simulink library "amg_sense_light_lib"  (R2015b)
settings: Solver=ode45  StartTime=0.0  StopTime=10.0  RelTol=1e-3
libraries: simulink x37, stm32f4_i2c_lib x3, waijung_soft_i2c_lib x3, waijung_customcode x1
(part 1 of 2)
settings Model: Creator=Krisada  LastModifiedBy=Aimagin
settings DataIOCC: SaveFormat=Array  SignalLoggingSaveFormat=ModelDataLogs
settings OptimizationCC: ExpressionDepthLimit=2147483647
settings DebuggingCC: UnderspecifiedInitializationDetection=Classic  MergeDetectMultiDrivingBlocksExec=none  SolverPrmCheckMsg=warning  FcnCallInpInsideContextMsg=UseLocalSettings  StateNameClashWarn=warning  StrictBusMsg=Warning
settings HardwareCC: ProdBitPerPointer=32  ProdLargestAtomicFloat=None  ProdIntDivRoundTo=Undefined  ProdEndianess=Unspecified  ProdWordSize=32  ProdHWDeviceType=32-bit Generic
settings GRTTargetCC: CombineOutputUpdateFcns=off  GRTInterface=on
settings ConfigComp: CovModelRefEnable=Off

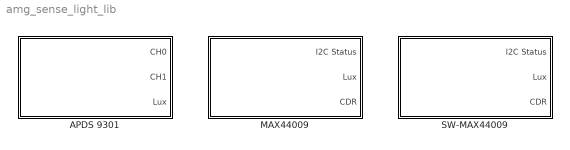
== system amg_sense_light_lib ==
  APDS 9301 : Subsystem  mask(stm32f4_i2c_sensors){module=1, slvaddr=hex2dec('72'), outputlabel={'CH0','CH1','Lux'}, sensorname=STM32F4\naMG Sense - Light, sampletime=0.5}
      mask prompts: module "I2C Module"; slvaddr "I2C Slave Address"; outputlabel "Output label"; sensorname "Sensor name"; sampletime "Sample time (sec)"
      mask help:
      | aMG Sense - Light
      |
      | Note: Require I2C Setup block for the selected I2C module.
      mask init:
      | stm32f4_i2c_sensors_callback('init');
      mask TypeOptions module: 1 | 2 | 3
      mask Callback module: stm32f4_i2c_sensors_callback('module');
      mask Display: text(0.5, 0.5, 'STM32F4\naMG Sense - Light','ver','middle','hor','center');port_label('output', 1,'CH0');port_label('output', 2,'CH1');port_label('output', 3,'Lux');
  MAX44009 : Subsystem  mask(stm32f4_i2c_sensors){module=1, slvaddr=hex2dec('94'), outputlabel={'I2C Status','Lux','CDR'}, sensorname=STM32F4\naMG Sense - Light\nMAX44009, sampletime=1}
      mask prompts: module "I2C Module"; slvaddr "I2C Slave Address"; outputlabel "Output label"; sensorname "Sensor name"; sampletime "Sample time (sec)"
      mask help:
      | aMG Sense - Light
      |
      | I2C Status:
      |  0 - Success
      |  1 - NAK
      |  2 - Timeout
      |  3 - Combined error, NAK+Timeout
      |
      | Note: Require I2C Setup block for the selected I2C module.
      mask init:
      | stm32f4_i2c_sensors_callback('init');
      mask TypeOptions module: 1 | 2 | 3
      mask Callback module: stm32f4_i2c_sensors_callback('module');
      mask Display: text(0.5, 0.5, 'STM32F4\naMG Sense - Light\nMAX44009','ver','middle','hor','center');port_label('output', 1,'I2C Status');port_label('output', 2,'Lux');port_label('output', 3,'CDR');
  SW-MAX44009 : Subsystem  mask(waijung_soft_i2c_sensors){module=1, slvaddr=hex2dec('94'), outputlabel={'I2C Status','Lux','CDR'}, sensorname=Soft-I2C\naMG Sense - Light\nMAX44009, sampletime=1}
      mask prompts: module "I2C Module"; slvaddr "I2C Slave Address"; outputlabel "Output label"; sensorname "Sensor name"; sampletime "Sample time (sec)"
      mask help:
      | aMG Sense - Light
      |
      | I2C Status:
      |  0 - Success
      |  1 - NAK
      |  2 - Timeout
      |  3 - Combined error, NAK+Timeout
      |
      | Note: Require I2C Setup block for the selected I2C module.
      mask init:
      | waijung_soft_i2c_sensors_callback('init');
      mask TypeOptions module: 1 | 2 | 3
      mask Callback module: waijung_soft_i2c_sensors_callback('module');
      mask Display: text(0.5, 0.5, 'Soft-I2C\naMG Sense - Light\nMAX44009','ver','middle','hor','center');port_label('output', 1,'I2C Status');port_label('output', 2,'Lux');port_label('output', 3,'CDR');

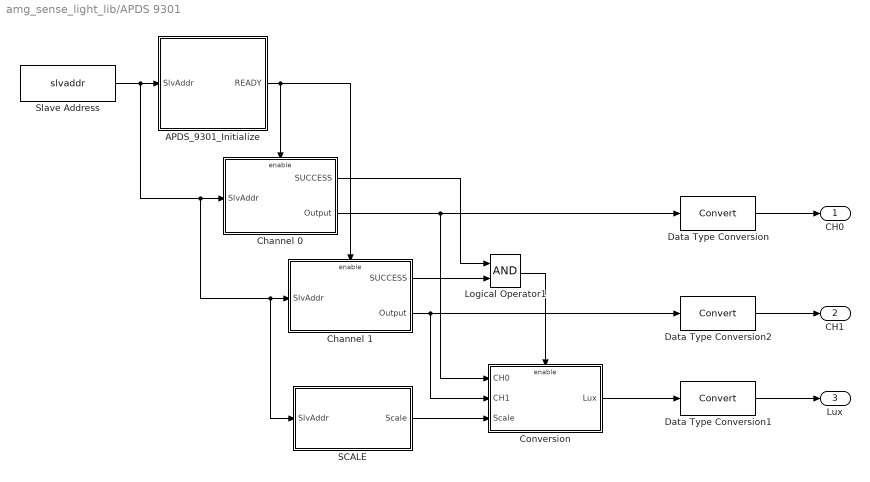
== system amg_sense_light_lib/APDS 9301 ==
  APDS_9301_Initialize : Subsystem
  Channel 0 : Subsystem
  Channel 1 : Subsystem
  Conversion : Subsystem
  Data Type Conversion : DataTypeConversion
  Data Type Conversion1 : DataTypeConversion
  Data Type Conversion2 : DataTypeConversion
  Logical Operator1 : Logic  AllPortsSameDT=off  OutDataTypeStr=boolean
  SCALE : Subsystem
  Slave Address : Constant  Value=slvaddr  OutDataTypeStr=uint8  SampleTime=sampletime
  CH0 : Outport
  CH1 : Outport  Port=2
  Lux : Outport  Port=3
  wires:
  Data Type Conversion/1 -> CH0/1
  Data Type Conversion2/1 -> CH1/1
  Data Type Conversion1/1 -> Lux/1
  Slave Address/1 -> APDS_9301_Initialize/1(SlvAddr), Channel 0/1(SlvAddr), Channel 1/1(SlvAddr), SCALE/1(SlvAddr)
  APDS_9301_Initialize/1(READY) -> Channel 0/Enable, Channel 1/Enable
  Channel 0/2(Output) -> Conversion/1(CH0), Data Type Conversion/1
  Channel 1/1(SUCCESS) -> Logical Operator1/2
  Channel 0/1(SUCCESS) -> Logical Operator1/1
  Conversion/1(Lux) -> Data Type Conversion1/1
  Channel 1/2(Output) -> Conversion/2(CH1), Data Type Conversion2/1
  Logical Operator1/1 -> Conversion/Enable
  SCALE/1(Scale) -> Conversion/3(Scale)

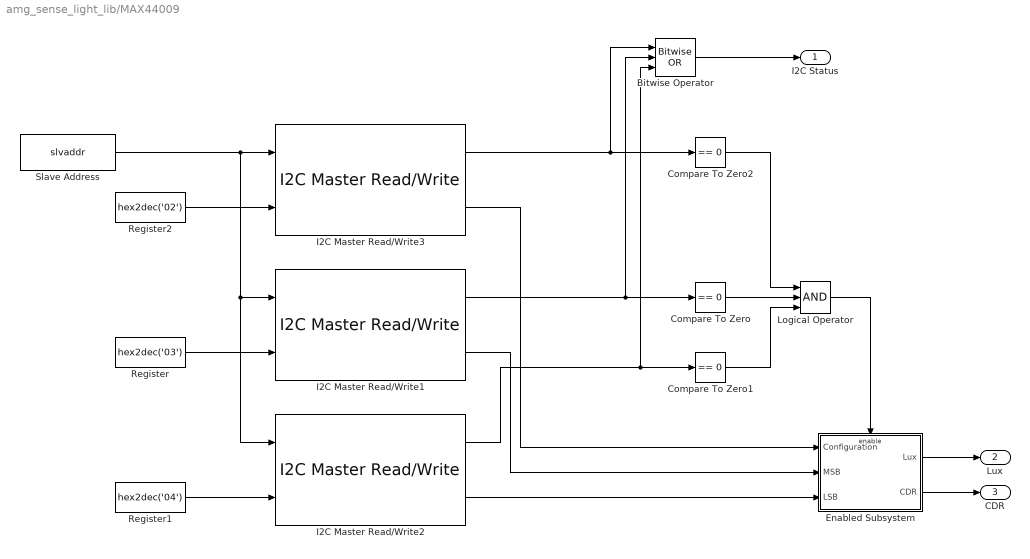
== system amg_sense_light_lib/MAX44009 ==
  Bitwise Operator : simulink/Logic and Bit Operations/Bitwise Operator  logicop=OR  UseBitMask=off  NumInputPorts=3  BitMask=bin2dec('11011001')  BitMaskRealWorld=Stored Integer
  Compare To Zero : simulink/Logic and Bit Operations/Compare To Zero  SystemSampleTime=-1  relop===  LogicOutDataTypeMode=uint8  ZeroCross=off
  Compare To Zero1 : simulink/Logic and Bit Operations/Compare To Zero  SystemSampleTime=-1  relop===  LogicOutDataTypeMode=uint8  ZeroCross=off
  Compare To Zero2 : simulink/Logic and Bit Operations/Compare To Zero  SystemSampleTime=-1  relop===  LogicOutDataTypeMode=uint8  ZeroCross=off
  Enabled Subsystem : Subsystem  TreatAsAtomicUnit=on
  I2C Master Read/Write1 : stm32f4_i2c_lib/I2C Master Read//Write  configuration=Transaction  module=1  lastmodule=3  transfer=Blocking  dutycycle=TLow/THigh = 2  clkspeed=400  timeout=25  writecount=1  readcount=1  sdapin=C9  sclpin=A8  waitwritetime=0  forcestop=off  inputtypearray=[2 3 3]  outputtypearray=[2 3 3]  confstr="[\"C\",\"9\",\"A\",\"8\",\"1\",\"1\",\"6\",\"0\",\"I2C_DutyCycle_2\",\"0\",\"off\"]"  sampletime=-1  sampletimestr=1  blockid=MAX44009I2CMasterReadWrite1
  I2C Master Read/Write2 : stm32f4_i2c_lib/I2C Master Read//Write  configuration=Transaction  module=1  lastmodule=3  transfer=Blocking  dutycycle=TLow/THigh = 2  clkspeed=400  timeout=25  writecount=1  readcount=1  sdapin=C9  sclpin=A8  waitwritetime=0  forcestop=off  inputtypearray=[2 3 3]  outputtypearray=[2 3 3]  confstr="[\"C\",\"9\",\"A\",\"8\",\"1\",\"1\",\"6\",\"0\",\"I2C_DutyCycle_2\",\"0\",\"off\"]"  sampletime=-1  sampletimestr=1  blockid=MAX44009I2CMasterReadWrite2
  I2C Master Read/Write3 : stm32f4_i2c_lib/I2C Master Read//Write  configuration=Transaction  module=1  lastmodule=3  transfer=Blocking  dutycycle=TLow/THigh = 2  clkspeed=400  timeout=25  writecount=1  readcount=1  sdapin=C9  sclpin=A8  waitwritetime=0  forcestop=off  inputtypearray=[2 3 3]  outputtypearray=[2 3 3]  confstr="[\"C\",\"9\",\"A\",\"8\",\"1\",\"1\",\"6\",\"0\",\"I2C_DutyCycle_2\",\"0\",\"off\"]"  sampletime=-1  sampletimestr=1  blockid=MAX44009I2CMasterReadWrite3
  Logical Operator : Logic  Inputs=3  AllPortsSameDT=off  OutDataTypeStr=boolean
  Register : Constant  Value=hex2dec('03')  OutDataTypeStr=uint8
  Register1 : Constant  Value=hex2dec('04')  OutDataTypeStr=uint8
  Register2 : Constant  Value=hex2dec('02')  OutDataTypeStr=uint8
  Slave Address : Constant  Value=slvaddr  OutDataTypeStr=uint8  SampleTime=sampletime
  I2C Status : Outport
  Lux : Outport  Port=2
  CDR : Outport  Port=3
  wires:
  I2C Master Read/Write3/2 -> Enabled Subsystem/1(Configuration)
  Compare To Zero1/1 -> Logical Operator/3
  Compare To Zero2/1 -> Logical Operator/1
  Compare To Zero/1 -> Logical Operator/2
  I2C Master Read/Write3/1 -> Compare To Zero2/1, Bitwise Operator/1
  Register2/1 -> I2C Master Read/Write3/2
  I2C Master Read/Write2/2 -> Enabled Subsystem/3(LSB)
  I2C Master Read/Write1/2 -> Enabled Subsystem/2(MSB)
  Logical Operator/1 -> Enabled Subsystem/Enable
  I2C Master Read/Write2/1 -> Compare To Zero1/1, Bitwise Operator/3
  Register1/1 -> I2C Master Read/Write2/2
  Slave Address/1 -> I2C Master Read/Write3/1, I2C Master Read/Write2/1, I2C Master Read/Write1/1
  Register/1 -> I2C Master Read/Write1/2
  I2C Master Read/Write1/1 -> Compare To Zero/1, Bitwise Operator/2
  Enabled Subsystem/1(Lux) -> Lux/1
  Enabled Subsystem/2(CDR) -> CDR/1
  Bitwise Operator/1 -> I2C Status/1

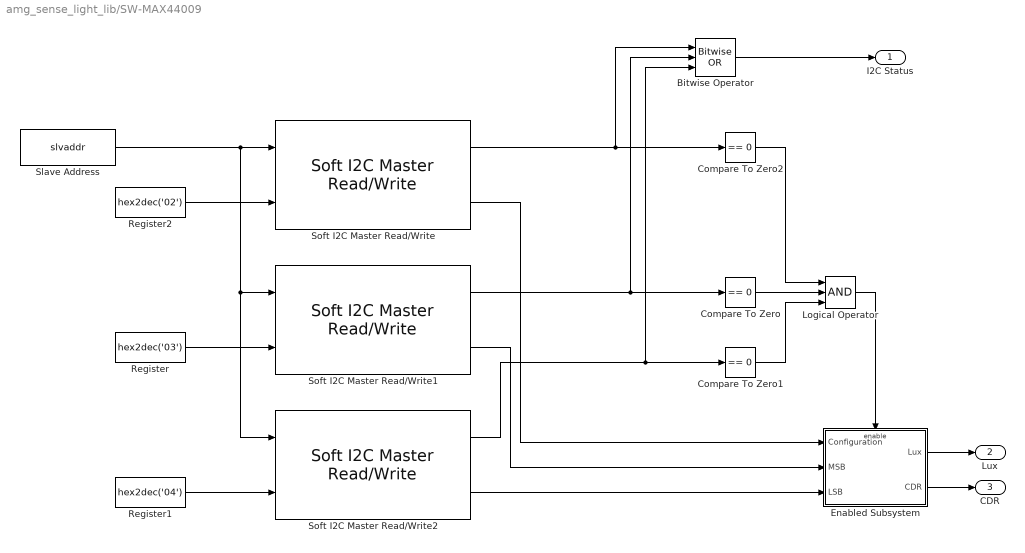
== system amg_sense_light_lib/SW-MAX44009 ==
  Bitwise Operator : simulink/Logic and Bit Operations/Bitwise Operator  logicop=OR  UseBitMask=off  NumInputPorts=3  BitMask=bin2dec('11011001')  BitMaskRealWorld=Stored Integer
  Compare To Zero : simulink/Logic and Bit Operations/Compare To Zero  SystemSampleTime=-1  relop===  LogicOutDataTypeMode=uint8  ZeroCross=off
  Compare To Zero1 : simulink/Logic and Bit Operations/Compare To Zero  SystemSampleTime=-1  relop===  LogicOutDataTypeMode=uint8  ZeroCross=off
  Compare To Zero2 : simulink/Logic and Bit Operations/Compare To Zero  SystemSampleTime=-1  relop===  LogicOutDataTypeMode=uint8  ZeroCross=off
  Enabled Subsystem : Subsystem  TreatAsAtomicUnit=on
  Logical Operator : Logic  Inputs=3  AllPortsSameDT=off  OutDataTypeStr=boolean
  Register : Constant  Value=hex2dec('03')  OutDataTypeStr=uint8
  Register1 : Constant  Value=hex2dec('04')  OutDataTypeStr=uint8
  Register2 : Constant  Value=hex2dec('02')  OutDataTypeStr=uint8
  Slave Address : Constant  Value=slvaddr  OutDataTypeStr=uint8  SampleTime=sampletime
  Soft I2C Master Read/Write : waijung_soft_i2c_lib/Soft I2C Master Read//Write  conf=ReadWrite  targetname=0  module=1  transfer=Blocking  clk=100  timeout=25  sdapins={'A4','A6'}  sclpins='A5'  writecount=1  readcount=1  waittime=0  forcestop=off  portpinstr=0  sampletime=inf  blockid=SWMAX44009SoftI2CMasterReadWrite  inputporttype=[3 3]  inputportwidth=[]  inputportlabel={'SlvAddr' 'Wr0 (uint8)'}  outputporttype=[3 3]  outputportwidth=[1 1]  outputportlabel={'Status' 'Rd0 (uint8)'}  compat=0  optionstring=[]
  Soft I2C Master Read/Write1 : waijung_soft_i2c_lib/Soft I2C Master Read//Write  conf=ReadWrite  targetname=0  module=1  transfer=Blocking  clk=100  timeout=25  sdapins={'A4','A6'}  sclpins='A5'  writecount=1  readcount=1  waittime=0  forcestop=off  portpinstr=0  sampletime=inf  blockid=SWMAX44009SoftI2CMasterReadWrite1  inputporttype=[3 3]  inputportwidth=[]  inputportlabel={'SlvAddr' 'Wr0 (uint8)'}  outputporttype=[3 3]  outputportwidth=[1 1]  outputportlabel={'Status' 'Rd0 (uint8)'}  compat=0  optionstring=[]
  Soft I2C Master Read/Write2 : waijung_soft_i2c_lib/Soft I2C Master Read//Write  conf=ReadWrite  targetname=0  module=1  transfer=Blocking  clk=100  timeout=25  sdapins={'A4','A6'}  sclpins='A5'  writecount=1  readcount=1  waittime=0  forcestop=off  portpinstr=0  sampletime=inf  blockid=SWMAX44009SoftI2CMasterReadWrite2  inputporttype=[3 3]  inputportwidth=[]  inputportlabel={'SlvAddr' 'Wr0 (uint8)'}  outputporttype=[3 3]  outputportwidth=[1 1]  outputportlabel={'Status' 'Rd0 (uint8)'}  compat=0  optionstring=[]
  I2C Status : Outport
  Lux : Outport  Port=2
  CDR : Outport  Port=3
  wires:
  Enabled Subsystem/2(CDR) -> CDR/1
  Enabled Subsystem/1(Lux) -> Lux/1
  Soft I2C Master Read/Write1/1 -> Compare To Zero/1, Bitwise Operator/2
  Register/1 -> Soft I2C Master Read/Write1/2
  Slave Address/1 -> Soft I2C Master Read/Write1/1, Soft I2C Master Read/Write2/1, Soft I2C Master Read/Write/1
  Register1/1 -> Soft I2C Master Read/Write2/2
  Soft I2C Master Read/Write2/1 -> Compare To Zero1/1, Bitwise Operator/3
  Logical Operator/1 -> Enabled Subsystem/Enable
  Soft I2C Master Read/Write1/2 -> Enabled Subsystem/2(MSB)
  Soft I2C Master Read/Write2/2 -> Enabled Subsystem/3(LSB)
  Register2/1 -> Soft I2C Master Read/Write/2
  Soft I2C Master Read/Write/1 -> Compare To Zero2/1, Bitwise Operator/1
  Compare To Zero/1 -> Logical Operator/2
  Compare To Zero2/1 -> Logical Operator/1
  Compare To Zero1/1 -> Logical Operator/3
  Soft I2C Master Read/Write/2 -> Enabled Subsystem/1(Configuration)
  Bitwise Operator/1 -> I2C Status/1

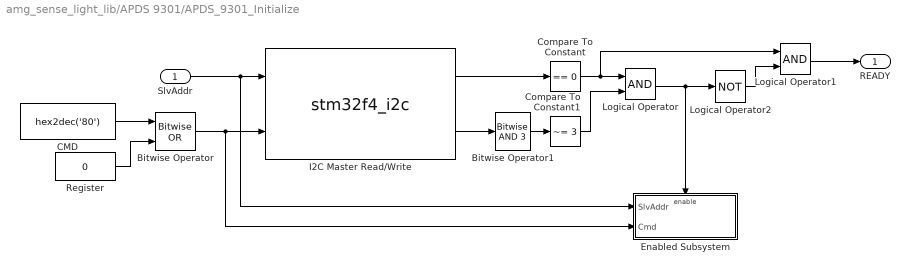
== system amg_sense_light_lib/APDS 9301/APDS_9301_Initialize ==
  SlvAddr : Inport
  Bitwise Operator : simulink/Logic and Bit Operations/Bitwise Operator  logicop=OR  UseBitMask=off  NumInputPorts=2  BitMask=bin2dec('11011001')  BitMaskRealWorld=Stored Integer
  Bitwise Operator1 : simulink/Logic and Bit Operations/Bitwise Operator  logicop=AND  UseBitMask=on  BitMask=3  BitMaskRealWorld=Stored Integer
  CMD : Constant  Value=hex2dec('80')  OutDataTypeStr=uint8
  Compare To Constant : simulink/Logic and Bit Operations/Compare To Constant  SystemSampleTime=-1  relop===  const=0  LogicOutDataTypeMode=uint8  ZeroCross=off
  Compare To Constant1 : simulink/Logic and Bit Operations/Compare To Constant  SystemSampleTime=-1  relop=~=  const=3  LogicOutDataTypeMode=uint8  ZeroCross=off
  Enabled Subsystem : Subsystem  TreatAsAtomicUnit=on
  I2C Master Read/Write : S-Function  FunctionName=stm32f4_i2c  Parameters=configuration,module,transfer,clkspeed,timeout,sdapin,sclpin,writecount,readcount,inputtypearray,outputtypearray,confstr,sampletime,sampletimestr,blockid  SFunctionDeploymentMode=off  EnableBusSupport=off  mask(stm32f4_i2c){configuration=Transaction, module=1, lastmodule=3, transfer=Blocking, dutycycle=TLow/THigh = 2, clkspeed=400, timeout=25, writecount=1, readcount=1, sdapin=C9, sclpin=A8, waitwritetime=0, inputtypearray=[2 3 3], outputtypearray=[2 3 3], confstr=["C","9","A","8","1","1","6","0","I2C_DutyCycle_2","0","off"], sampletime=-1, sampletimestr=1, blockid=APDS_9301_InitializeI2CMasterReadWrite}
      mask prompts: module "I2C Module"; lastmodule "Last module"; transfer "Transfer mode"; dutycycle "Duty cycle in fast mode"; clkspeed "Clock speed (kHz)"; timeout "Timeout (ms)"; writecount "Bytes write count"; readcount "Bytes read count"; sdapin "SDA pin"; sclpin "SCL pin"; waitwritetime "Wait write time (ms), default is 0"; inputtypearray "Input type array"; outputtypearray "Output type array"; confstr "Configuration string"; sampletime "Sample time (sec)"; sampletimestr "Compiled sample time (sec) in string"
      mask init:
      | stm32f4_i2c_callback('init');
      mask Help: web(fullfile(waijungdocroot,'stm32f4_i2c_readwrite.htm'), '-browser')
      mask TypeOptions configuration: Setup | Transaction
      mask Callback configuration: stm32f4_i2c_callback('configuration');
      mask TypeOptions module: 1 | 2 | 3
      mask Callback module: stm32f4_i2c_callback('module');
      mask TypeOptions transfer: Blocking | Non-blocking
      mask TypeOptions dutycycle: TLow/THigh = 16/9 | TLow/THigh = 2
      mask Callback dutycycle: stm32f4_i2c_callback('dutycycle');
      mask Callback writecount: stm32f4_i2c_callback('writecount');
      mask Callback readcount: stm32f4_i2c_callback('readcount');
      mask TypeOptions sdapin: - | C9
      mask Callback sdapin: stm32f4_i2c_callback('sdapin');
      mask TypeOptions sclpin: - | A8
      mask Callback sclpin: stm32f4_i2c_callback('sclpin');
      mask Callback confstr: stm32f4_i2c_callback('confstr');
      mask Callback sampletime: stm32f4_i2c_callback('sampletime');
      mask Callback sampletimestr: stm32f4_i2c_callback('sampletimestr');
      mask Callback blockid: stm32f4_i2c_callback('blockid');
      mask Display: text(0.5, 0.5, 'Module: I2C1\nTransfer: Blocking\nWrite: 1 bytes\nRead: 1 bytes\nTs (sec): 1','ver','middle','hor','center');port_label('input', 1,'SlvAddr');port_label('input', 2,'Wr0 (uint8)');port_label('output', 1,'Status');port_label('output', 2,'Rd0 (uint8)');
  Logical Operator : Logic  AllPortsSameDT=off  OutDataTypeStr=boolean
  Logical Operator1 : Logic  AllPortsSameDT=off  OutDataTypeStr=boolean
  Logical Operator2 : Logic  Operator=NOT  AllPortsSameDT=off  OutDataTypeStr=boolean
  Register : Constant  Value=0  OutDataTypeStr=uint8
  READY : Outport
  wires:
  SlvAddr/1 -> I2C Master Read/Write/1, Enabled Subsystem/1(SlvAddr)
  Bitwise Operator/1 -> I2C Master Read/Write/2, Enabled Subsystem/2(Cmd)
  CMD/1 -> Bitwise Operator/1
  I2C Master Read/Write/1 -> Compare To Constant/1
  I2C Master Read/Write/2 -> Bitwise Operator1/1
  Compare To Constant/1 -> Logical Operator/1, Logical Operator1/1
  Compare To Constant1/1 -> Logical Operator/2
  Logical Operator/1 -> Enabled Subsystem/Enable, Logical Operator2/1
  Register/1 -> Bitwise Operator/2
  Bitwise Operator1/1 -> Compare To Constant1/1
  Logical Operator2/1 -> Logical Operator1/2
  Logical Operator1/1 -> READY/1

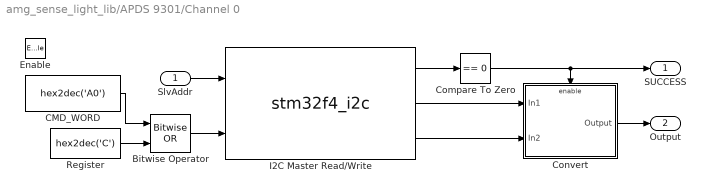
== system amg_sense_light_lib/APDS 9301/Channel 0 ==
  SlvAddr : Inport
  Enable : EnablePort  PropagateVarSize=During execution
  Bitwise Operator : simulink/Logic and Bit Operations/Bitwise Operator  logicop=OR  UseBitMask=off  NumInputPorts=2  BitMask=bin2dec('11011001')  BitMaskRealWorld=Stored Integer
  CMD_WORD : Constant  Value=hex2dec('A0')  OutDataTypeStr=uint8
  Compare To Zero : simulink/Logic and Bit Operations/Compare To Zero  SystemSampleTime=-1  relop===  LogicOutDataTypeMode=uint8  ZeroCross=off
  Convert : Subsystem
  I2C Master Read/Write : S-Function  FunctionName=stm32f4_i2c  Parameters=configuration,module,transfer,clkspeed,timeout,sdapin,sclpin,writecount,readcount,inputtypearray,outputtypearray,confstr,sampletime,sampletimestr,blockid  SFunctionDeploymentMode=off  EnableBusSupport=off  mask(stm32f4_i2c){configuration=Transaction, module=1, lastmodule=3, transfer=Blocking, dutycycle=TLow/THigh = 2, clkspeed=400, timeout=25, writecount=1, readcount=2, sdapin=C9, sclpin=A8, waitwritetime=0, inputtypearray=[2 3 3], outputtypearray=[3 3 3 3], confstr=["C","9","A","8","1","1","6","0","I2C_DutyCycle_2","0","off"], sampletime=-1, sampletimestr=1, blockid=Channel0I2CMasterReadWrite}
      mask prompts: module "I2C Module"; lastmodule "Last module"; transfer "Transfer mode"; dutycycle "Duty cycle in fast mode"; clkspeed "Clock speed (kHz)"; timeout "Timeout (ms)"; writecount "Bytes write count"; readcount "Bytes read count"; sdapin "SDA pin"; sclpin "SCL pin"; waitwritetime "Wait write time (ms), default is 0"; inputtypearray "Input type array"; outputtypearray "Output type array"; confstr "Configuration string"; sampletime "Sample time (sec)"; sampletimestr "Compiled sample time (sec) in string"
      mask init:
      | stm32f4_i2c_callback('init');
      mask Help: web(fullfile(waijungdocroot,'stm32f4_i2c_readwrite.htm'), '-browser')
      mask TypeOptions configuration: Setup | Transaction
      mask Callback configuration: stm32f4_i2c_callback('configuration');
      mask TypeOptions module: 1 | 2 | 3
      mask Callback module: stm32f4_i2c_callback('module');
      mask TypeOptions transfer: Blocking | Non-blocking
      mask TypeOptions dutycycle: TLow/THigh = 16/9 | TLow/THigh = 2
      mask Callback dutycycle: stm32f4_i2c_callback('dutycycle');
      mask Callback writecount: stm32f4_i2c_callback('writecount');
      mask Callback readcount: stm32f4_i2c_callback('readcount');
      mask TypeOptions sdapin: - | C9
      mask Callback sdapin: stm32f4_i2c_callback('sdapin');
      mask TypeOptions sclpin: - | A8
      mask Callback sclpin: stm32f4_i2c_callback('sclpin');
      mask Callback confstr: stm32f4_i2c_callback('confstr');
      mask Callback sampletime: stm32f4_i2c_callback('sampletime');
      mask Callback sampletimestr: stm32f4_i2c_callback('sampletimestr');
      mask Callback blockid: stm32f4_i2c_callback('blockid');
      mask Display: text(0.5, 0.5, 'Module: I2C1\nTransfer: Blocking\nWrite: 1 bytes\nRead: 2 bytes\nTs (sec): 1','ver','middle','hor','center');port_label('input', 1,'SlvAddr');port_label('input', 2,'Wr0 (uint8)');port_label('output', 1,'Status');port_label('output', 2,'Rd0 (uint8)');port_label('output', 3,'Rd1 (uint8)');
  Register : Constant  Value=hex2dec('C')  OutDataTypeStr=uint8
  SUCCESS : Outport
  Output : Outport  Port=2
  wires:
  SlvAddr/1 -> I2C Master Read/Write/1
  Bitwise Operator/1 -> I2C Master Read/Write/2
  CMD_WORD/1 -> Bitwise Operator/1
  Register/1 -> Bitwise Operator/2
  I2C Master Read/Write/2 -> Convert/1(In1)
  I2C Master Read/Write/3 -> Convert/2(In2)
  I2C Master Read/Write/1 -> Compare To Zero/1
  Convert/1(Output) -> Output/1
  Compare To Zero/1 -> SUCCESS/1, Convert/Enable

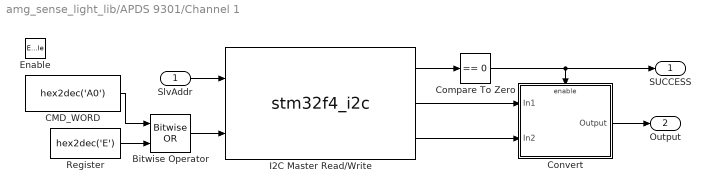
== system amg_sense_light_lib/APDS 9301/Channel 1 ==
  SlvAddr : Inport
  Enable : EnablePort  PropagateVarSize=During execution
  Bitwise Operator : simulink/Logic and Bit Operations/Bitwise Operator  logicop=OR  UseBitMask=off  NumInputPorts=2  BitMask=bin2dec('11011001')  BitMaskRealWorld=Stored Integer
  CMD_WORD : Constant  Value=hex2dec('A0')  OutDataTypeStr=uint8
  Compare To Zero : simulink/Logic and Bit Operations/Compare To Zero  SystemSampleTime=-1  relop===  LogicOutDataTypeMode=uint8  ZeroCross=off
  Convert : Subsystem
  I2C Master Read/Write : S-Function  FunctionName=stm32f4_i2c  Parameters=configuration,module,transfer,clkspeed,timeout,sdapin,sclpin,writecount,readcount,inputtypearray,outputtypearray,confstr,sampletime,sampletimestr,blockid  SFunctionDeploymentMode=off  EnableBusSupport=off  mask(stm32f4_i2c){configuration=Transaction, module=1, lastmodule=3, transfer=Blocking, dutycycle=TLow/THigh = 2, clkspeed=400, timeout=25, writecount=1, readcount=2, sdapin=C9, sclpin=A8, waitwritetime=0, inputtypearray=[2 3 3], outputtypearray=[3 3 3 3], confstr=["C","9","A","8","1","1","6","0","I2C_DutyCycle_2","0","off"], sampletime=-1, sampletimestr=1, blockid=Channel1I2CMasterReadWrite}
      mask prompts: module "I2C Module"; lastmodule "Last module"; transfer "Transfer mode"; dutycycle "Duty cycle in fast mode"; clkspeed "Clock speed (kHz)"; timeout "Timeout (ms)"; writecount "Bytes write count"; readcount "Bytes read count"; sdapin "SDA pin"; sclpin "SCL pin"; waitwritetime "Wait write time (ms), default is 0"; inputtypearray "Input type array"; outputtypearray "Output type array"; confstr "Configuration string"; sampletime "Sample time (sec)"; sampletimestr "Compiled sample time (sec) in string"
      mask init:
      | stm32f4_i2c_callback('init');
      mask Help: web(fullfile(waijungdocroot,'stm32f4_i2c_readwrite.htm'), '-browser')
      mask TypeOptions configuration: Setup | Transaction
      mask Callback configuration: stm32f4_i2c_callback('configuration');
      mask TypeOptions module: 1 | 2 | 3
      mask Callback module: stm32f4_i2c_callback('module');
      mask TypeOptions transfer: Blocking | Non-blocking
      mask TypeOptions dutycycle: TLow/THigh = 16/9 | TLow/THigh = 2
      mask Callback dutycycle: stm32f4_i2c_callback('dutycycle');
      mask Callback writecount: stm32f4_i2c_callback('writecount');
      mask Callback readcount: stm32f4_i2c_callback('readcount');
      mask TypeOptions sdapin: - | C9
      mask Callback sdapin: stm32f4_i2c_callback('sdapin');
      mask TypeOptions sclpin: - | A8
      mask Callback sclpin: stm32f4_i2c_callback('sclpin');
      mask Callback confstr: stm32f4_i2c_callback('confstr');
      mask Callback sampletime: stm32f4_i2c_callback('sampletime');
      mask Callback sampletimestr: stm32f4_i2c_callback('sampletimestr');
      mask Callback blockid: stm32f4_i2c_callback('blockid');
      mask Display: text(0.5, 0.5, 'Module: I2C1\nTransfer: Blocking\nWrite: 1 bytes\nRead: 2 bytes\nTs (sec): 1','ver','middle','hor','center');port_label('input', 1,'SlvAddr');port_label('input', 2,'Wr0 (uint8)');port_label('output', 1,'Status');port_label('output', 2,'Rd0 (uint8)');port_label('output', 3,'Rd1 (uint8)');
  Register : Constant  Value=hex2dec('E')  OutDataTypeStr=uint8
  SUCCESS : Outport
  Output : Outport  Port=2
  wires:
  Convert/1(Output) -> Output/1
  Compare To Zero/1 -> SUCCESS/1, Convert/Enable
  I2C Master Read/Write/1 -> Compare To Zero/1
  I2C Master Read/Write/3 -> Convert/2(In2)
  I2C Master Read/Write/2 -> Convert/1(In1)
  Register/1 -> Bitwise Operator/2
  CMD_WORD/1 -> Bitwise Operator/1
  Bitwise Operator/1 -> I2C Master Read/Write/2
  SlvAddr/1 -> I2C Master Read/Write/1

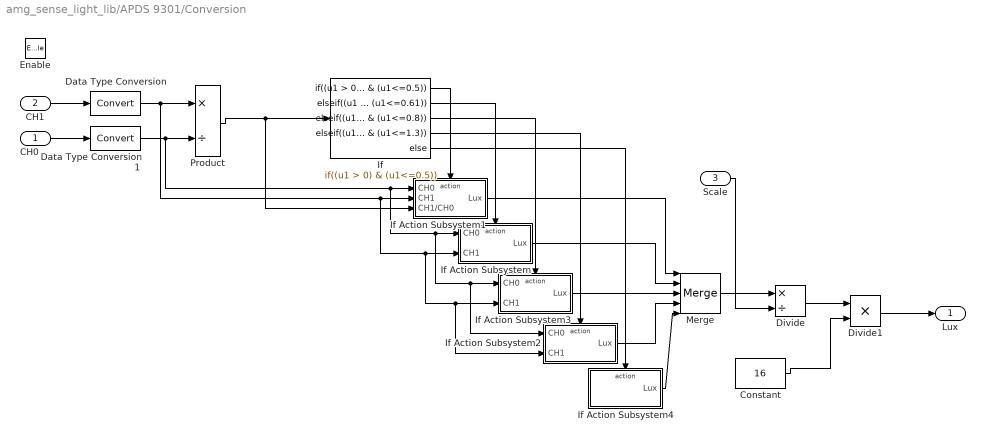
== system amg_sense_light_lib/APDS 9301/Conversion ==
  CH0 : Inport
  CH1 : Inport  Port=2
  Scale : Inport  Port=3
  Enable : EnablePort  PropagateVarSize=During execution
  Constant : Constant  Value=16
  Data Type Conversion : DataTypeConversion
  Data Type Conversion1 : DataTypeConversion
  Divide : Product  Inputs=*/
  Divide1 : Product  Inputs=**
  If : If  IfExpression=(u1 > 0) & (u1<=0.5)  ElseIfExpressions=(u1 > 0.5) & (u1<=0.61),(u1 > 0.61) & (u1<=0.8),(u1 > 0.8) & (u1<=1.3)
  If Action Subsystem : Subsystem  TreatAsAtomicUnit=on
  If Action Subsystem1 : Subsystem  TreatAsAtomicUnit=on
  If Action Subsystem2 : Subsystem  TreatAsAtomicUnit=on
  If Action Subsystem3 : Subsystem  TreatAsAtomicUnit=on
  If Action Subsystem4 : Subsystem  TreatAsAtomicUnit=on
  Merge : Merge  Inputs=5
  Product : Product  Inputs=*/  RndMeth=Zero
  Lux : Outport
  wires:
  CH1/1 -> Data Type Conversion/1
  CH0/1 -> Data Type Conversion1/1
  Product/1 -> If/1, If Action Subsystem1/3(CH1/CH0)
  If/1 -> If Action Subsystem1/Action
  If/2 -> If Action Subsystem/Action
  If/3 -> If Action Subsystem3/Action
  If/4 -> If Action Subsystem2/Action
  If/5 -> If Action Subsystem4/Action
  Data Type Conversion/1 -> Product/1, If Action Subsystem1/2(CH1), If Action Subsystem/2(CH1), If Action Subsystem3/2(CH1), If Action Subsystem2/2(CH1)
  Data Type Conversion1/1 -> Product/2, If Action Subsystem1/1(CH0), If Action Subsystem/1(CH0), If Action Subsystem3/1(CH0), If Action Subsystem2/1(CH0)
  Scale/1 -> Divide/2
  Divide/1 -> Divide1/1
  Constant/1 -> Divide1/2
  Divide1/1 -> Lux/1
  If Action Subsystem1/1(Lux) -> Merge/1
  If Action Subsystem/1(Lux) -> Merge/2
  If Action Subsystem3/1(Lux) -> Merge/3
  If Action Subsystem2/1(Lux) -> Merge/4
  If Action Subsystem4/1(Lux) -> Merge/5
  Merge/1 -> Divide/1

== system amg_sense_light_lib/APDS 9301/SCALE ==
  note: # Priority: 0
  SlvAddr : Inport
  Constant : Constant  Value=hex2dec('02')  OutDataTypeStr=uint8
  Subsystem : Subsystem
  Subsystem1 : Subsystem
  Terminator : Terminator
  Scale : Outport
  wires:
  SlvAddr/1 -> Subsystem/1(SlvAddr), Subsystem1/1(SlvAddr)
  Subsystem/1(READY) -> Terminator/1
  Subsystem1/1(Conf_scale) -> Scale/1
  Constant/1 -> Subsystem/2(Value)

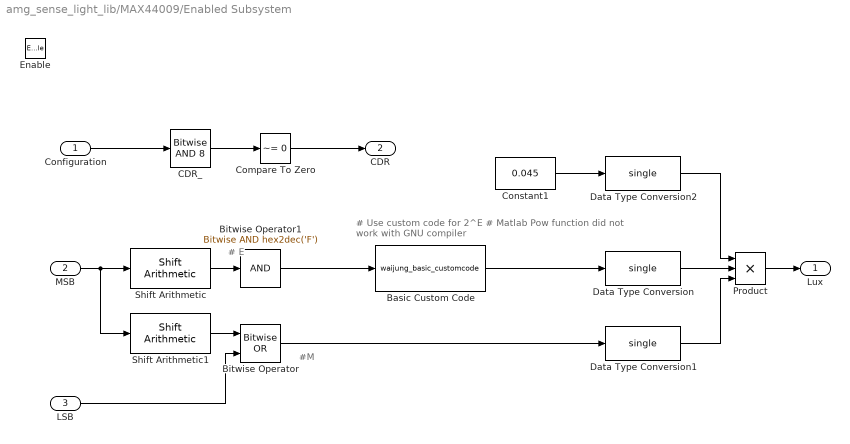
== system amg_sense_light_lib/MAX44009/Enabled Subsystem ==
  note: #M
  note: # E
  note: # Use custom code for 2^E
      | # Matlab Pow function did not work with GNU compiler
  Configuration : Inport
  MSB : Inport  Port=2
  LSB : Inport  Port=3
  Enable : EnablePort  PropagateVarSize=During execution
  Basic Custom Code : S-Function  FunctionName=waijung_basic_customcode  Parameters=inputportcount,inputporttypeid,outputportcount,outputporttypeid,sampletime,blockid,cinputportlabelstr,coutputportlabelstr,incfilestrarray,outputporttype,inputporttype,initialfuncallstr,enablefuncallstr,outputfuncallstr,disablefuncallstr,inputportdiminfo,outputportdiminfo  SFunctionDeploymentMode=off  EnableBusSupport=off  mask(waijung_basic_customcode){inputporttype=uint8, cinputportlabel=E, cinputportlabelstr=["E"], inputportcount=1, inputporttypeid=[3], outputporttype=uint32, coutputportlabel=2^E, coutputportlabelstr=["2^E"], outputportcount=1, outputporttypeid=[7], incpath={}, srcpath={}, incfiles={}, srcfiles={}, initialfuncallstr=, enablefuncallstr=, outputfuncallstr={uint32_T result = 1; uint8_T i; for (i=0; i<in1; i++) { result *= 2; } *out1 = result;}, disablefuncallstr=, sampletime=inf, sampletimestr=0, blockid=MAX44009EnabledSubsystemBasicCustomCode, enablecustomportlabel=on, incfilestrarray=[], inputportdiminfo=[1  1  1  3], outputportdiminfo=[1  1  1  7]}
      mask prompts: inputporttype "Input port definition (data type) separted by comma e.g. double, single, double, uint8"; cinputportlabel "Custom input port labels (Ex. In1, In2, In3)"; cinputportlabelstr "Custom input port type string"; inputportcount "Input port count"; inputporttypeid "Input port data type ID"; outputporttype "Output port definition  (data type) separted by comma e.g. double, single, double, uint8"; coutputportlabel "Custom output port labels (Ex. Out1, Out2, Out3)"; coutputportlabelstr "Custom output port type string"; outputportcount "Output port count"; outputporttypeid "Output port data type ID"; incpath "Path for include files (*.h), defined as cell array of string."; srcpath "Path for source files (*.c), defined as cell array of string."; incfiles "Included header file names with extension (.h), defined as cell array of string."; srcfiles "Included source file names with extension (.c), defined as cell array of string."; initialfuncallstr "Initial function call string"; enablefuncallstr "Enable function call string"; outputfuncallstr "Output function call string"; disablefuncallstr "Disable function call string"; sampletime "Sample time (sec)"; sampletimestr "Sample time string"; blockid "Block ID"; enablecustomportlabel "Enable custom port labels"; incfilestrarray "Header file array"; inputportdiminfo "Input Port Dimension Information (Define in cmex)"; outputportdiminfo "Output Port Dimension Information"
      mask help:
      | This block implements a basic custom code block.
      |
      | Allowed input/output datatype:
      | dynamic,double,single,int8,uint8,int16,uint16,int32,uint32,boolean. Leave this field empty if no input or output needed.
      |
      | "Path for include files" defines the include path. All *.h files in these path(s) will be used in the build process.
      |
      | "Path for source files" defines path to look for each source file(s) defined in the "Included source file name ...". All required source file(s) and source file path(s) must be explicitly defined.
      |
      | "Included header file names ..." field is used to list any *.h file that will be included in #include statements of waijung_hwdrvlib.h.
      |
      | The Basic Custom Code Block supports 2-D input/output matrix/vector signals.
      |
      | The dimensions of input signals are automatically inherited from the supplied input signals.
      | The dimensions of output signals must be implicitly defined using the following format.
      |
      | DataType:nRowsxnCols
      |
      | If dimensions are not defined, scalar signal (1x1) is assumed.
      |
      | For examples: double:4x5,int8,int16:3x1
      mask init:
      | waijung_basic_customcode_callback('init');
      mask Help: web(fullfile(waijungdocroot,'waijung_basic_customcode.htm'), '-browser')
      mask Callback inputporttype: waijung_basic_customcode_callback('inputporttype');
      mask Callback cinputportlabel: waijung_basic_customcode_callback('cinputportlabel');
      mask Callback outputporttype: waijung_basic_customcode_callback('outputporttype');
      mask Callback coutputportlabel: waijung_basic_customcode_callback('coutputportlabel');
      mask Callback incfiles: waijung_basic_customcode_callback('incfiles');
      mask Callback sampletime: waijung_basic_customcode_callback('sampletime');
      mask Callback blockid: waijung_basic_customcode_callback('blockid');
      mask Display: text(0.5, 0.5, 'Ts (sec): 0','ver','middle','hor','center');port_label('input', 1,'E');port_label('output', 1,'2^E')
  Bitwise Operator : simulink/Logic and Bit Operations/Bitwise Operator  logicop=OR  UseBitMask=off  NumInputPorts=2  BitMask=bin2dec('11011001')  BitMaskRealWorld=Stored Integer
  Bitwise Operator1 : simulink/Logic and Bit Operations/Bitwise Operator  logicop=AND  UseBitMask=on  BitMask=hex2dec('F')  BitMaskRealWorld=Stored Integer
  CDR_ : simulink/Logic and Bit Operations/Bitwise Operator  logicop=AND  UseBitMask=on  BitMask=8  BitMaskRealWorld=Stored Integer
  Compare To Zero : simulink/Logic and Bit Operations/Compare To Zero  SystemSampleTime=-1  relop=~=  LogicOutDataTypeMode=uint8  ZeroCross=off
  Constant1 : Constant  Value=0.045
  Data Type Conversion : DataTypeConversion  OutDataTypeStr=single
  Data Type Conversion1 : DataTypeConversion  OutDataTypeStr=single
  Data Type Conversion2 : DataTypeConversion  OutDataTypeStr=single
  Product : Product  Inputs=3  RndMeth=Zero  OutDataTypeStr=Inherit: Same as first input
  Shift Arithmetic : simulink/Logic and Bit Operations/Shift Arithmetic  SystemSampleTime=-1  nBitShiftRight=4  nBinPtShiftRight=0
  Shift Arithmetic1 : simulink/Logic and Bit Operations/Shift Arithmetic  SystemSampleTime=-1  nBitShiftRight=-4  nBinPtShiftRight=0
  Lux : Outport
  CDR : Outport  Port=2
  wires:
  Product/1 -> Lux/1
  Configuration/1 -> CDR_/1
  Data Type Conversion1/1 -> Product/3
  Bitwise Operator/1 -> Data Type Conversion1/1
  LSB/1 -> Bitwise Operator/2
  Shift Arithmetic1/1 -> Bitwise Operator/1
  Shift Arithmetic/1 -> Bitwise Operator1/1
  MSB/1 -> Shift Arithmetic1/1, Shift Arithmetic/1
  Basic Custom Code/1 -> Data Type Conversion/1
  Constant1/1 -> Data Type Conversion2/1
  Bitwise Operator1/1 -> Basic Custom Code/1
  Data Type Conversion/1 -> Product/2
  Data Type Conversion2/1 -> Product/1
  CDR_/1 -> Compare To Zero/1
  Compare To Zero/1 -> CDR/1

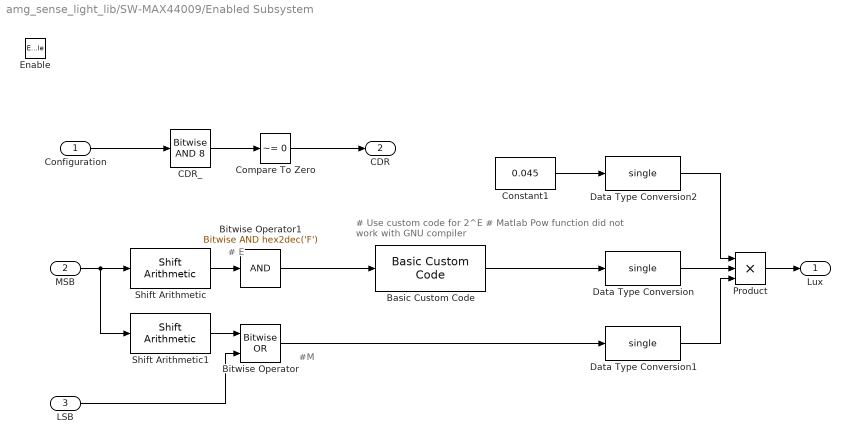
== system amg_sense_light_lib/SW-MAX44009/Enabled Subsystem ==
  note: # Use custom code for 2^E
      | # Matlab Pow function did not work with GNU compiler
  note: # E
  note: #M
  Configuration : Inport
  MSB : Inport  Port=2
  LSB : Inport  Port=3
  Enable : EnablePort  PropagateVarSize=During execution
  Basic Custom Code : waijung_customcode/Basic Custom Code  inputporttype=uint8  cinputportlabel=E  cinputportlabelstr="[\"E\"]"  inputportcount=1  inputporttypeid=[3]  outputporttype=uint32  coutputportlabel=2^E  coutputportlabelstr="[\"2^E\"]"  outputportcount=1  outputporttypeid=[7]  incpath={}  srcpath={}  incfiles={}  srcfiles={}  outputfuncallstr={uint32_T result = 1; uint8_T i; for (i=0; i<in1; i++) { result *= 2; } *out1 = result;}  sampletime=inf  sampletimestr=0  blockid=SWMAX44009EnabledSubsystemBasicCustomCode  enablecustomportlabel=on  incfilestrarray=[]  inputportdiminfo="[1  1  1  3]"  outputportdiminfo="[1  1  1  7]"
  Bitwise Operator : simulink/Logic and Bit Operations/Bitwise Operator  logicop=OR  UseBitMask=off  NumInputPorts=2  BitMask=bin2dec('11011001')  BitMaskRealWorld=Stored Integer
  Bitwise Operator1 : simulink/Logic and Bit Operations/Bitwise Operator  logicop=AND  UseBitMask=on  BitMask=hex2dec('F')  BitMaskRealWorld=Stored Integer
  CDR_ : simulink/Logic and Bit Operations/Bitwise Operator  logicop=AND  UseBitMask=on  BitMask=8  BitMaskRealWorld=Stored Integer
  Compare To Zero : simulink/Logic and Bit Operations/Compare To Zero  SystemSampleTime=-1  relop=~=  LogicOutDataTypeMode=uint8  ZeroCross=off
  Constant1 : Constant  Value=0.045
  Data Type Conversion : DataTypeConversion  OutDataTypeStr=single
  Data Type Conversion1 : DataTypeConversion  OutDataTypeStr=single
  Data Type Conversion2 : DataTypeConversion  OutDataTypeStr=single
  Product : Product  Inputs=3  RndMeth=Zero  OutDataTypeStr=Inherit: Same as first input
  Shift Arithmetic : simulink/Logic and Bit Operations/Shift Arithmetic  SystemSampleTime=-1  nBitShiftRight=4  nBinPtShiftRight=0
  Shift Arithmetic1 : simulink/Logic and Bit Operations/Shift Arithmetic  SystemSampleTime=-1  nBitShiftRight=-4  nBinPtShiftRight=0
  Lux : Outport
  CDR : Outport  Port=2
  wires:
  Compare To Zero/1 -> CDR/1
  CDR_/1 -> Compare To Zero/1
  Data Type Conversion2/1 -> Product/1
  Data Type Conversion/1 -> Product/2
  Bitwise Operator1/1 -> Basic Custom Code/1
  Constant1/1 -> Data Type Conversion2/1
  Basic Custom Code/1 -> Data Type Conversion/1
  MSB/1 -> Shift Arithmetic/1, Shift Arithmetic1/1
  Shift Arithmetic/1 -> Bitwise Operator1/1
  Shift Arithmetic1/1 -> Bitwise Operator/1
  LSB/1 -> Bitwise Operator/2
  Bitwise Operator/1 -> Data Type Conversion1/1
  Data Type Conversion1/1 -> Product/3
  Configuration/1 -> CDR_/1
  Product/1 -> Lux/1

== system amg_sense_light_lib/APDS 9301/APDS_9301_Initialize/Enabled Subsystem ==
  SlvAddr : Inport
  Cmd : Inport  Port=2
  Enable : EnablePort  PropagateVarSize=During execution
  I2C Master Read/Write : S-Function  FunctionName=stm32f4_i2c  Parameters=configuration,module,transfer,clkspeed,timeout,sdapin,sclpin,writecount,readcount,inputtypearray,outputtypearray,confstr,sampletime,sampletimestr,blockid  SFunctionDeploymentMode=off  EnableBusSupport=off  mask(stm32f4_i2c){configuration=Transaction, module=1, lastmodule=3, transfer=Blocking, dutycycle=TLow/THigh = 2, clkspeed=400, timeout=25, writecount=2, readcount=0, sdapin=C9, sclpin=A8, waitwritetime=0, inputtypearray=[3 3 3 3], outputtypearray=[1 3], confstr=["C","9","A","8","1","1","6","0","I2C_DutyCycle_2","0","off"], sampletime=-1, sampletimestr=1, blockid=APDS_9301_InitializeEnabledSubsystemI2CMasterReadWrite}
      mask prompts: module "I2C Module"; lastmodule "Last module"; transfer "Transfer mode"; dutycycle "Duty cycle in fast mode"; clkspeed "Clock speed (kHz)"; timeout "Timeout (ms)"; writecount "Bytes write count"; readcount "Bytes read count"; sdapin "SDA pin"; sclpin "SCL pin"; waitwritetime "Wait write time (ms), default is 0"; inputtypearray "Input type array"; outputtypearray "Output type array"; confstr "Configuration string"; sampletime "Sample time (sec)"; sampletimestr "Compiled sample time (sec) in string"
      mask init:
      | stm32f4_i2c_callback('init');
      mask Help: web(fullfile(waijungdocroot,'stm32f4_i2c_readwrite.htm'), '-browser')
      mask TypeOptions configuration: Setup | Transaction
      mask Callback configuration: stm32f4_i2c_callback('configuration');
      mask TypeOptions module: 1 | 2 | 3
      mask Callback module: stm32f4_i2c_callback('module');
      mask TypeOptions transfer: Blocking | Non-blocking
      mask TypeOptions dutycycle: TLow/THigh = 16/9 | TLow/THigh = 2
      mask Callback dutycycle: stm32f4_i2c_callback('dutycycle');
      mask Callback writecount: stm32f4_i2c_callback('writecount');
      mask Callback readcount: stm32f4_i2c_callback('readcount');
      mask TypeOptions sdapin: - | C9
      mask Callback sdapin: stm32f4_i2c_callback('sdapin');
      mask TypeOptions sclpin: - | A8
      mask Callback sclpin: stm32f4_i2c_callback('sclpin');
      mask Callback confstr: stm32f4_i2c_callback('confstr');
      mask Callback sampletime: stm32f4_i2c_callback('sampletime');
      mask Callback sampletimestr: stm32f4_i2c_callback('sampletimestr');
      mask Callback blockid: stm32f4_i2c_callback('blockid');
      mask Display: text(0.5, 0.5, 'Module: I2C1\nTransfer: Blocking\nWrite: 2 bytes\nRead: 0 bytes\nTs (sec): 1','ver','middle','hor','center');port_label('input', 1,'SlvAddr');port_label('input', 2,'Wr0 (uint8)');port_label('input', 3,'Wr1 (uint8)');port_label('output', 1,'Status');
  Power ON : Constant  Value=3  OutDataTypeStr=uint8
  Terminator : Terminator
  wires:
  SlvAddr/1 -> I2C Master Read/Write/1
  Cmd/1 -> I2C Master Read/Write/2
  Power ON/1 -> I2C Master Read/Write/3
  I2C Master Read/Write/1 -> Terminator/1

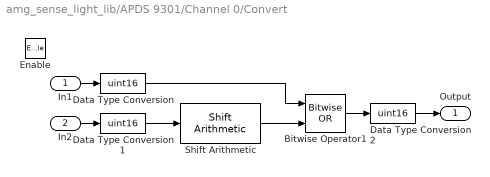
== system amg_sense_light_lib/APDS 9301/Channel 0/Convert ==
  In1 : Inport
  In2 : Inport  Port=2
  Enable : EnablePort  PropagateVarSize=During execution
  Bitwise Operator1 : simulink/Logic and Bit Operations/Bitwise Operator  logicop=OR  UseBitMask=off  NumInputPorts=2  BitMask=bin2dec('11011001')  BitMaskRealWorld=Stored Integer
  Data Type Conversion : DataTypeConversion  OutDataTypeStr=uint16
  Data Type Conversion1 : DataTypeConversion  OutDataTypeStr=uint16
  Data Type Conversion2 : DataTypeConversion  OutDataTypeStr=uint16
  Shift Arithmetic : simulink/Logic and Bit Operations/Shift Arithmetic  SystemSampleTime=-1  nBitShiftRight=-8  nBinPtShiftRight=0
  Output : Outport
  wires:
  Shift Arithmetic/1 -> Bitwise Operator1/2
  Bitwise Operator1/1 -> Data Type Conversion2/1
  In1/1 -> Data Type Conversion/1
  Data Type Conversion2/1 -> Output/1
  In2/1 -> Data Type Conversion1/1
  Data Type Conversion1/1 -> Shift Arithmetic/1
  Data Type Conversion/1 -> Bitwise Operator1/1

== system amg_sense_light_lib/APDS 9301/Channel 1/Convert ==
  In1 : Inport
  In2 : Inport  Port=2
  Enable : EnablePort  PropagateVarSize=During execution
  Bitwise Operator1 : simulink/Logic and Bit Operations/Bitwise Operator  logicop=OR  UseBitMask=off  NumInputPorts=2  BitMask=bin2dec('11011001')  BitMaskRealWorld=Stored Integer
  Data Type Conversion : DataTypeConversion  OutDataTypeStr=uint16
  Data Type Conversion1 : DataTypeConversion  OutDataTypeStr=uint16
  Data Type Conversion2 : DataTypeConversion  OutDataTypeStr=uint16
  Shift Arithmetic : simulink/Logic and Bit Operations/Shift Arithmetic  SystemSampleTime=-1  nBitShiftRight=-8  nBinPtShiftRight=0
  Output : Outport
  wires:
  Data Type Conversion/1 -> Bitwise Operator1/1
  Data Type Conversion1/1 -> Shift Arithmetic/1
  In2/1 -> Data Type Conversion1/1
  Data Type Conversion2/1 -> Output/1
  In1/1 -> Data Type Conversion/1
  Bitwise Operator1/1 -> Data Type Conversion2/1
  Shift Arithmetic/1 -> Bitwise Operator1/2

== system amg_sense_light_lib/APDS 9301/Conversion/If Action Subsystem ==
  CH0 : Inport
  CH1 : Inport  Port=2
  Action Port : ActionPort  PropagateVarSize=During execution
  Gain : Gain  Gain=0.0224
  Gain1 : Gain  Gain=0.031
  Subtract : Sum  Inputs=+-
  Lux : Outport
  wires:
  CH0/1 -> Gain/1
  Subtract/1 -> Lux/1
  CH1/1 -> Gain1/1
  Gain/1 -> Subtract/1
  Gain1/1 -> Subtract/2

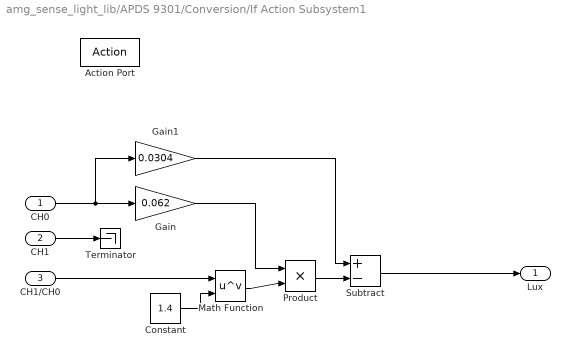
== system amg_sense_light_lib/APDS 9301/Conversion/If Action Subsystem1 ==
  CH0 : Inport
  CH1 : Inport  Port=2
  CH1/CH0 : Inport  Port=3
  Action Port : ActionPort  PropagateVarSize=During execution
  Constant : Constant  Value=1.4
  Gain : Gain  Gain=0.062
  Gain1 : Gain  Gain=0.0304
  Math Function : Math  Operator=pow  SaturateOnIntegerOverflow=on
  Product : Product  RndMeth=Zero
  Subtract : Sum  Inputs=+-
  Terminator : Terminator
  Lux : Outport
  wires:
  CH0/1 -> Gain/1, Gain1/1
  Constant/1 -> Math Function/2
  CH1/CH0/1 -> Math Function/1
  Gain/1 -> Product/1
  Math Function/1 -> Product/2
  Gain1/1 -> Subtract/1
  Product/1 -> Subtract/2
  Subtract/1 -> Lux/1
  CH1/1 -> Terminator/1

== system amg_sense_light_lib/APDS 9301/Conversion/If Action Subsystem2 ==
  CH0 : Inport
  CH1 : Inport  Port=2
  Action Port : ActionPort  PropagateVarSize=During execution
  Gain : Gain  Gain=0.00146
  Gain1 : Gain  Gain=0.00112
  Subtract : Sum  Inputs=+-
  Lux : Outport
  wires:
  CH0/1 -> Gain/1
  Subtract/1 -> Lux/1
  CH1/1 -> Gain1/1
  Gain/1 -> Subtract/1
  Gain1/1 -> Subtract/2

== system amg_sense_light_lib/APDS 9301/Conversion/If Action Subsystem3 ==
  CH0 : Inport
  CH1 : Inport  Port=2
  Action Port : ActionPort  PropagateVarSize=During execution
  Gain : Gain  Gain=0.0128
  Gain1 : Gain  Gain=0.0153
  Subtract : Sum  Inputs=+-
  Lux : Outport
  wires:
  CH0/1 -> Gain/1
  Subtract/1 -> Lux/1
  CH1/1 -> Gain1/1
  Gain/1 -> Subtract/1
  Gain1/1 -> Subtract/2

== system amg_sense_light_lib/APDS 9301/Conversion/If Action Subsystem4 ==
  Action Port : ActionPort  PropagateVarSize=During execution
  Constant : Constant  Value=0
  Lux : Outport
  wires:
  Constant/1 -> Lux/1

== system amg_sense_light_lib/APDS 9301/SCALE/Subsystem ==
  SlvAddr : Inport
  Value : Inport  Port=2
  Bitwise Operator2 : simulink/Logic and Bit Operations/Bitwise Operator  logicop=OR  UseBitMask=off  NumInputPorts=2  BitMask=bin2dec('11011001')  BitMaskRealWorld=Stored Integer
  CMD1 : Constant  Value=hex2dec('80')  OutDataTypeStr=uint8
  Compare To Zero : simulink/Logic and Bit Operations/Compare To Zero  SystemSampleTime=-1  relop===  LogicOutDataTypeMode=uint8  ZeroCross=off
  I2C Master Read/Write : S-Function  FunctionName=stm32f4_i2c  Parameters=configuration,module,transfer,clkspeed,timeout,sdapin,sclpin,writecount,readcount,inputtypearray,outputtypearray,confstr,sampletime,sampletimestr,blockid  SFunctionDeploymentMode=off  EnableBusSupport=off  mask(stm32f4_i2c){configuration=Transaction, module=1, lastmodule=3, transfer=Blocking, dutycycle=TLow/THigh = 2, clkspeed=400, timeout=25, writecount=2, readcount=0, sdapin=C9, sclpin=A8, waitwritetime=0, inputtypearray=[3 3 3 3], outputtypearray=[1 3], confstr=["C","9","A","8","1","1","6","0","I2C_DutyCycle_2","0","off"], sampletime=-1, sampletimestr=1, blockid=SCALESubsystemI2CMasterReadWrite}
      mask prompts: module "I2C Module"; lastmodule "Last module"; transfer "Transfer mode"; dutycycle "Duty cycle in fast mode"; clkspeed "Clock speed (kHz)"; timeout "Timeout (ms)"; writecount "Bytes write count"; readcount "Bytes read count"; sdapin "SDA pin"; sclpin "SCL pin"; waitwritetime "Wait write time (ms), default is 0"; inputtypearray "Input type array"; outputtypearray "Output type array"; confstr "Configuration string"; sampletime "Sample time (sec)"; sampletimestr "Compiled sample time (sec) in string"
      mask init:
      | stm32f4_i2c_callback('init');
      mask Help: web(fullfile(waijungdocroot,'stm32f4_i2c_readwrite.htm'), '-browser')
      mask TypeOptions configuration: Setup | Transaction
      mask Callback configuration: stm32f4_i2c_callback('configuration');
      mask TypeOptions module: 1 | 2 | 3
      mask Callback module: stm32f4_i2c_callback('module');
      mask TypeOptions transfer: Blocking | Non-blocking
      mask TypeOptions dutycycle: TLow/THigh = 16/9 | TLow/THigh = 2
      mask Callback dutycycle: stm32f4_i2c_callback('dutycycle');
      mask Callback writecount: stm32f4_i2c_callback('writecount');
      mask Callback readcount: stm32f4_i2c_callback('readcount');
      mask TypeOptions sdapin: - | C9
      mask Callback sdapin: stm32f4_i2c_callback('sdapin');
      mask TypeOptions sclpin: - | A8
      mask Callback sclpin: stm32f4_i2c_callback('sclpin');
      mask Callback confstr: stm32f4_i2c_callback('confstr');
      mask Callback sampletime: stm32f4_i2c_callback('sampletime');
      mask Callback sampletimestr: stm32f4_i2c_callback('sampletimestr');
      mask Callback blockid: stm32f4_i2c_callback('blockid');
      mask Display: text(0.5, 0.5, 'Module: I2C1\nTransfer: Blocking\nWrite: 2 bytes\nRead: 0 bytes\nTs (sec): 1','ver','middle','hor','center');port_label('input', 1,'SlvAddr');port_label('input', 2,'Wr0 (uint8)');port_label('input', 3,'Wr1 (uint8)');port_label('output', 1,'Status');
  Register1 : Constant  OutDataTypeStr=uint8
  READY : Outport
  wires:
  SlvAddr/1 -> I2C Master Read/Write/1
  Value/1 -> I2C Master Read/Write/3
  CMD1/1 -> Bitwise Operator2/1
  Register1/1 -> Bitwise Operator2/2
  Bitwise Operator2/1 -> I2C Master Read/Write/2
  I2C Master Read/Write/1 -> Compare To Zero/1
  Compare To Zero/1 -> READY/1

== system amg_sense_light_lib/APDS 9301/SCALE/Subsystem1 ==
  SlvAddr : Inport
  Bitwise Operator2 : simulink/Logic and Bit Operations/Bitwise Operator  logicop=OR  UseBitMask=off  NumInputPorts=2  BitMask=bin2dec('11011001')  BitMaskRealWorld=Stored Integer
  CMD1 : Constant  Value=hex2dec('80')  OutDataTypeStr=uint8
  Compare To Zero : simulink/Logic and Bit Operations/Compare To Zero  SystemSampleTime=-1  relop===  LogicOutDataTypeMode=uint8  ZeroCross=off
  I2C Master Read/Write : S-Function  Priority=0  FunctionName=stm32f4_i2c  Parameters=configuration,module,transfer,clkspeed,timeout,sdapin,sclpin,writecount,readcount,inputtypearray,outputtypearray,confstr,sampletime,sampletimestr,blockid  SFunctionDeploymentMode=off  EnableBusSupport=off  mask(stm32f4_i2c){configuration=Transaction, module=1, lastmodule=3, transfer=Blocking, dutycycle=TLow/THigh = 2, clkspeed=400, timeout=25, writecount=1, readcount=1, sdapin=C9, sclpin=A8, waitwritetime=0, inputtypearray=[2 3 3], outputtypearray=[2 3 3], confstr=["C","9","A","8","1","1","6","0","I2C_DutyCycle_2","0","off"], sampletime=-1, sampletimestr=1, blockid=SCALESubsystem1I2CMasterReadWrite}
      mask prompts: module "I2C Module"; lastmodule "Last module"; transfer "Transfer mode"; dutycycle "Duty cycle in fast mode"; clkspeed "Clock speed (kHz)"; timeout "Timeout (ms)"; writecount "Bytes write count"; readcount "Bytes read count"; sdapin "SDA pin"; sclpin "SCL pin"; waitwritetime "Wait write time (ms), default is 0"; inputtypearray "Input type array"; outputtypearray "Output type array"; confstr "Configuration string"; sampletime "Sample time (sec)"; sampletimestr "Compiled sample time (sec) in string"
      mask init:
      | stm32f4_i2c_callback('init');
      mask Help: web(fullfile(waijungdocroot,'stm32f4_i2c_readwrite.htm'), '-browser')
      mask TypeOptions configuration: Setup | Transaction
      mask Callback configuration: stm32f4_i2c_callback('configuration');
      mask TypeOptions module: 1 | 2 | 3
      mask Callback module: stm32f4_i2c_callback('module');
      mask TypeOptions transfer: Blocking | Non-blocking
      mask TypeOptions dutycycle: TLow/THigh = 16/9 | TLow/THigh = 2
      mask Callback dutycycle: stm32f4_i2c_callback('dutycycle');
      mask Callback writecount: stm32f4_i2c_callback('writecount');
      mask Callback readcount: stm32f4_i2c_callback('readcount');
      mask TypeOptions sdapin: - | C9
      mask Callback sdapin: stm32f4_i2c_callback('sdapin');
      mask TypeOptions sclpin: - | A8
      mask Callback sclpin: stm32f4_i2c_callback('sclpin');
      mask Callback confstr: stm32f4_i2c_callback('confstr');
      mask Callback sampletime: stm32f4_i2c_callback('sampletime');
      mask Callback sampletimestr: stm32f4_i2c_callback('sampletimestr');
      mask Callback blockid: stm32f4_i2c_callback('blockid');
      mask Display: text(0.5, 0.5, 'Module: I2C1\nTransfer: Blocking\nWrite: 1 bytes\nRead: 1 bytes\nTs (sec): 1','ver','middle','hor','center');port_label('input', 1,'SlvAddr');port_label('input', 2,'Wr0 (uint8)');port_label('output', 1,'Status');port_label('output', 2,'Rd0 (uint8)');
  Register1 : Constant  OutDataTypeStr=uint8
  Subsystem : Subsystem
  Conf_scale : Outport
  wires:
  Compare To Zero/1 -> Subsystem/Enable
  I2C Master Read/Write/1 -> Compare To Zero/1
  Bitwise Operator2/1 -> I2C Master Read/Write/2
  Register1/1 -> Bitwise Operator2/2
  CMD1/1 -> Bitwise Operator2/1
  SlvAddr/1 -> I2C Master Read/Write/1
  I2C Master Read/Write/2 -> Subsystem/1(In1)
  Subsystem/1(Out1) -> Conf_scale/1
